simulink model "Mechanical_Accelerometer"  (R2023b)
settings: Solver=VariableStepAuto  StartTime=0.0  StopTime=50  MaxStep=0.01  RelTol=1e-3
model workspace (MAT data in the model file):
  M = 10
  Ms = 100
  b = 12
  k = 32
settings Model: Creator=91839  LastModifiedBy=siva kumar
settings SolverCC: AlgebraicLoopSolver=TrustRegion
settings DataIOCC: ExternalInput=data  SaveFormat=Array  DSMLogging=off  ReturnWorkspaceOutputs=off
settings DebuggingCC: UnconnectedInputMsg=warning  UnconnectedOutputMsg=warning  UnconnectedLineMsg=warning
settings ModelReferenceCC: EnableRefExpFcnMdlSchedulingChecks=on
settings SFSimCC: CustomCodeUndefinedFunction=UseInterfaceOnly

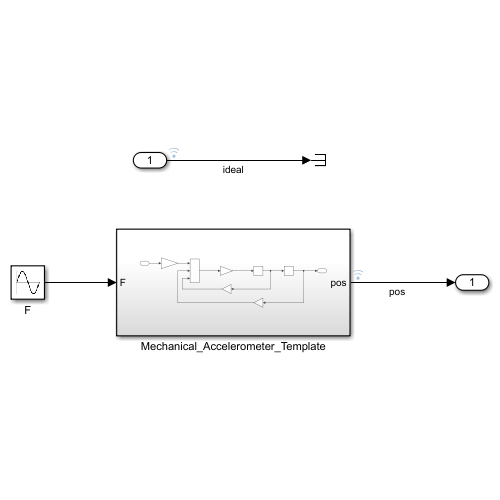
[thumbnail: Simulink's stored preview of the top-level diagram]
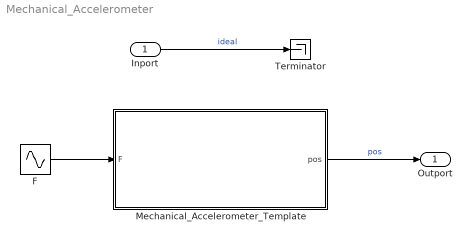
== system Mechanical_Accelerometer ==
  Inport : Inport
  F : Sin  Amplitude=3  SampleTime=0
  Mechanical_Accelerometer_Template : Subsystem
  Terminator : Terminator
  Outport : Outport
  wires:
  Inport/1 -> Terminator/1  "ideal"
  F/1 -> Mechanical_Accelerometer_Template/1(F)
  Mechanical_Accelerometer_Template/1(pos) -> Outport/1  "pos"

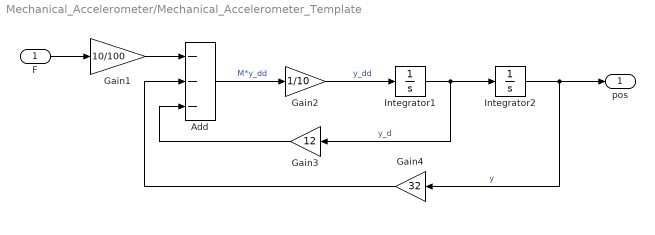
== system Mechanical_Accelerometer/Mechanical_Accelerometer_Template ==
  F : Inport
  Add : Sum  Inputs=---
  Gain1 : Gain  Gain=10/100
  Gain2 : Gain  Gain=1/10
  Gain3 : Gain  Gain=12
  Gain4 : Gain  Gain=32
  Integrator1 : Integrator
  Integrator2 : Integrator
  pos : Outport
  wires:
  Gain3/1 -> Add/3
  Integrator2/1 -> pos/1, Gain4/1  "y"
  Gain4/1 -> Add/2
  Gain1/1 -> Add/1
  Gain2/1 -> Integrator1/1  "y_dd"
  Integrator1/1 -> Integrator2/1, Gain3/1  "y_d"
  Add/1 -> Gain2/1  "M*y_dd"
  F/1 -> Gain1/1
